simulink model "Model_Comparison_mks_landinglinear"  (R2022b)
settings: Solver=VariableStepAuto  StartTime=0.0  StopTime=4500  FixedStep=0.5  RelTol=1e-6
settings Model: Creator=Mitarbeiter  LastModifiedBy=Mitarbeiter

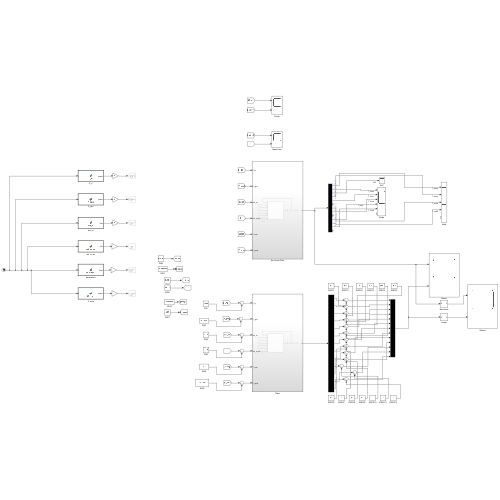
[thumbnail: Simulink's stored preview of the top-level diagram]
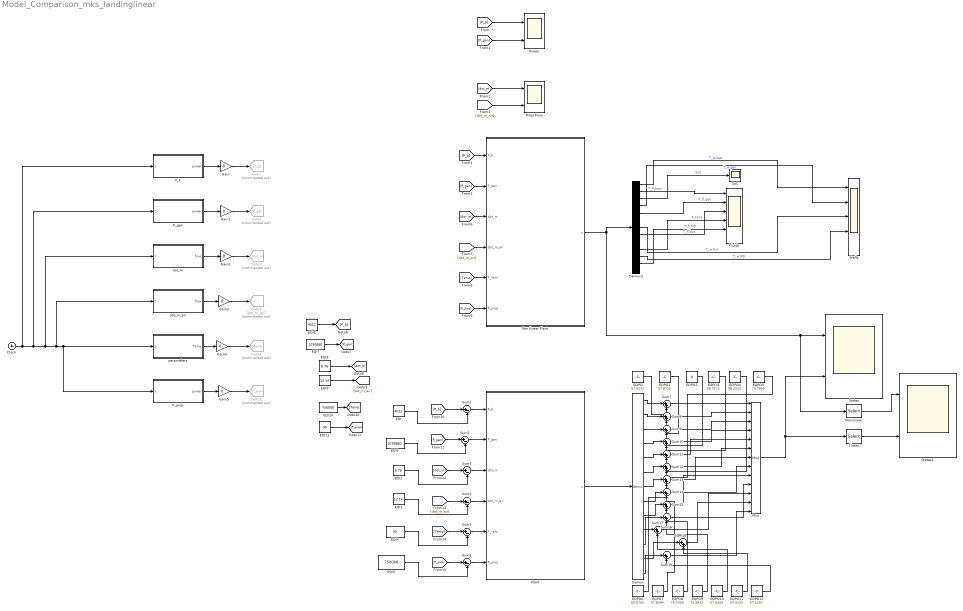
== system Model_Comparison_mks_landinglinear ==
  Clock : Clock
  Demux : Demux  Outputs=13
  Demux1 : Demux  Outputs=13
  EQI : Constant  Value=4012
  EQI1 : Constant  Value=1076880
  EQI10 : Constant  Value=750000
  EQI11 : Constant  Value=30
  EQI2 : Constant  Value=6.76
  EQI3 : Constant  Value=12.14
  EQI4 : Constant  Value=30
  EQI5 : Constant  Value=750000
  EQI6 : Constant  Value=4012
  EQI7 : Constant  Value=1076880
  EQI8 : Constant  Value=6.76
  EQI9 : Constant  Value=12.14
  EQPO : Constant  Value=57.9131
  EQPO1 : Constant  Value=57.8725
  EQPO10 : Constant  Value=57.8394
  EQPO11 : Constant  Value=57.3135
  EQPO12 : Constant  Value=57.1297
  EQPO2 : Constant  Value=0
  EQPO3 : Constant  Value=58.7172
  EQPO4 : Constant  Value=58.2512
  EQPO5 : Constant  Value=74.7995
  EQPO6 : Constant  Value=65.6701
  EQPO7 : Constant  Value=57.8394
  EQPO8 : Constant  Value=76.7055
  EQPO9 : Constant  Value=71.8433
  Fluids : Scope  NumInputPorts=6
  Gain{,1..5} (6 alike) : Gain  Gain=0
  Goto : Goto  Commented=on  GotoTag=P_b
  Goto1 : Goto  Commented=on  GotoTag=P_gen
  Goto2 : Goto  Commented=on  GotoTag=dot_m
  Goto3 : Goto  Commented=on  GotoTag=dot_m_air
  Goto4 : Goto  Commented=on  GotoTag=Temp
  Goto5 : Goto  Commented=on  GotoTag=P_prop
  Linear : Selector  InputPortWidth=13  IndexOptions=Index vector (dialog)  Indices=[1 2 3 4 5 6 7 8 9 10]  OutputSizes=1
  Mass Flow : Scope  NumInputPorts=2
  Mux : Mux  Inputs=13
  Non linear Plant : Subsystem
  Non-linear : Selector  InputPortWidth=13  IndexOptions=Index vector (dialog)  Indices=[1 2 3 4 5 6 7 8 9 10]  OutputSizes=1
  P_b : MATLAB Function  TreatAsAtomicUnit=on
  P_gen : MATLAB Function  TreatAsAtomicUnit=on
  P_prop : MATLAB Function  TreatAsAtomicUnit=on
  Plant : Subsystem
  Power : Scope  NumInputPorts=2
  SoC : Scope
  States : Scope  NumInputPorts=2
  States1 : Scope  NumInputPorts=2
  Sum{1..6} (6 alike) : Sum  Inputs=|+-
  Sum{7..19} (13 alike) : Sum  Inputs=|++
  Walls : Scope  NumInputPorts=5
  dot_m : MATLAB Function  TreatAsAtomicUnit=on
  dot_m_air : MATLAB Function  TreatAsAtomicUnit=on
  parameters : MATLAB Function  TreatAsAtomicUnit=on
  wires:
  Clock/1 -> P_b/1(t), P_gen/1(t), dot_m/1(t), dot_m_air/1(t), parameters/1(t), P_prop/1(t)
  Non linear Plant/1(x) -> Demux1/1, Non-linear/1, States/1
  Demux1/3 -> SoC/1  "SoC"
  Demux1/1 -> Walls/1  "T_w,batt"
  Demux1/2 -> Fluids/1  "T_fl,batt"
  Demux1/4 -> Walls/2  "T_w,gen"
  Demux1/5 -> Fluids/2  "T_fl,gen"
  Demux1/7 -> Walls/3  "T_w,bus"
  Demux1/8 -> Fluids/3  "T_fl,bus"
  Demux1/10 -> Fluids/4  "T_tank"
  Demux1/12 -> Fluids/5  "T_fl,MD"
  Demux1/11 -> Walls/4  "T_w,MD"
  dot_m/1(flow) -> Gain2/1
  P_gen/1(power) -> Gain1/1
  Plant/1(x) -> Demux/1
  Mux/1 -> States/2, Linear/1
  Non-linear/1 -> States1/1
  Linear/1 -> States1/2
  dot_m_air/1(flow) -> Gain3/1
  [P_b] -> Power/1
  [P_gen] -> Power/2
  [dot_m] -> Mass Flow/1
  [dot_m_air] -> Mass Flow/2
  P_b/1(power) -> Gain/1
  [P_b] -> Non linear Plant/1(P_b)
  [P_gen] -> Non linear Plant/2(P_gen)
  [dot_m] -> Non linear Plant/3(dot_m)
  [dot_m_air] -> Non linear Plant/4(dot_m_air)
  parameters/1(Temp) -> Gain4/1
  P_prop/1(power) -> Gain5/1
  [Temp] -> Non linear Plant/5(T_ram)
  [P_prop] -> Non linear Plant/6(P_prop)
  Sum2/1 -> Plant/1(P_b)
  [P_b] -> Sum2/1
  Sum1/1 -> Plant/2(P_gen)
  [dot_m] -> Sum3/1
  [P_gen] -> Sum1/1
  [dot_m_air] -> Sum4/1
  [Temp] -> Sum5/1
  [P_prop] -> Sum6/1
  Sum3/1 -> Plant/3(dot_m)
  Sum4/1 -> Plant/4(dot_m_air)
  Sum5/1 -> Plant/5(T_ram)
  Sum6/1 -> Plant/6(P_prop)
  EQI1/1 -> Sum1/2
  EQI/1 -> Sum2/2
  EQI2/1 -> Sum3/2
  EQI3/1 -> Sum4/2
  EQI4/1 -> Sum5/2
  EQI5/1 -> Sum6/2
  Demux/1 -> Sum7/1
  Demux/2 -> Sum8/1
  Demux/3 -> Sum9/1
  Demux/4 -> Sum10/1
  Demux/5 -> Sum11/1
  Demux/6 -> Sum12/1
  Demux/7 -> Sum13/1
  Demux/8 -> Sum14/1
  Demux/9 -> Sum15/1
  Demux/10 -> Sum16/1
  Demux/11 -> Sum17/1
  Demux/12 -> Sum18/1
  Demux/13 -> Sum19/1
  Sum7/1 -> Mux/1
  Sum8/1 -> Mux/2
  Sum9/1 -> Mux/3
  Sum10/1 -> Mux/4
  Sum11/1 -> Mux/5
  Sum12/1 -> Mux/6
  Sum13/1 -> Mux/7
  Sum14/1 -> Mux/8
  Sum15/1 -> Mux/9
  Sum16/1 -> Mux/10
  Sum17/1 -> Mux/11
  Sum18/1 -> Mux/12
  Sum19/1 -> Mux/13
  EQPO/1 -> Sum7/2
  EQPO1/1 -> Sum8/2
  EQPO2/1 -> Sum9/2
  EQPO3/1 -> Sum10/2
  EQPO4/1 -> Sum11/2
  EQPO5/1 -> Sum12/2
  EQPO6/1 -> Sum13/2
  EQPO7/1 -> Sum14/2
  EQPO8/1 -> Sum15/2
  EQPO9/1 -> Sum16/2
  EQPO10/1 -> Sum17/2
  EQPO11/1 -> Sum18/2
  EQPO12/1 -> Sum19/2
  Gain/1 -> Goto/1
  Gain1/1 -> Goto1/1
  Gain2/1 -> Goto2/1
  Gain3/1 -> Goto3/1
  Gain4/1 -> Goto4/1
  Gain5/1 -> Goto5/1
  EQI6/1 -> [P_b]
  EQI7/1 -> [P_gen]
  EQI8/1 -> [dot_m]
  EQI9/1 -> [dot_m_air]
  EQI10/1 -> [Temp]
  EQI11/1 -> [P_prop]

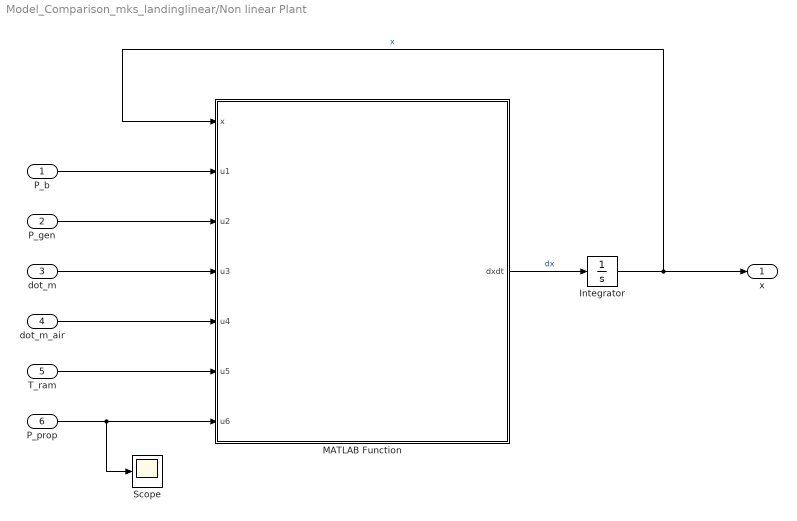
== system Model_Comparison_mks_landinglinear/Non linear Plant ==
  P_b : Inport
  P_gen : Inport  Port=2
  dot_m : Inport  Port=3
  dot_m_air : Inport  Port=4
  T_ram : Inport  Port=5
  P_prop : Inport  Port=6
  Integrator : Integrator  InitialCondition=[57.913; 57.872; 0; 58.717; 58.251; 74.799; 65.670; 57.839; 76.705; 71.843; 57.839; 57.313; 57.130]
  MATLAB Function : MATLAB Function  TreatAsAtomicUnit=on
  Scope : Scope
  x : Outport
  wires:
  MATLAB Function/1(dxdt) -> Integrator/1  "dx"
  Integrator/1 -> x/1, MATLAB Function/1(x)  "x"
  P_prop/1 -> Scope/1, MATLAB Function/7(u6)
  P_b/1 -> MATLAB Function/2(u1)
  P_gen/1 -> MATLAB Function/3(u2)
  dot_m/1 -> MATLAB Function/4(u3)
  dot_m_air/1 -> MATLAB Function/5(u4)
  T_ram/1 -> MATLAB Function/6(u5)

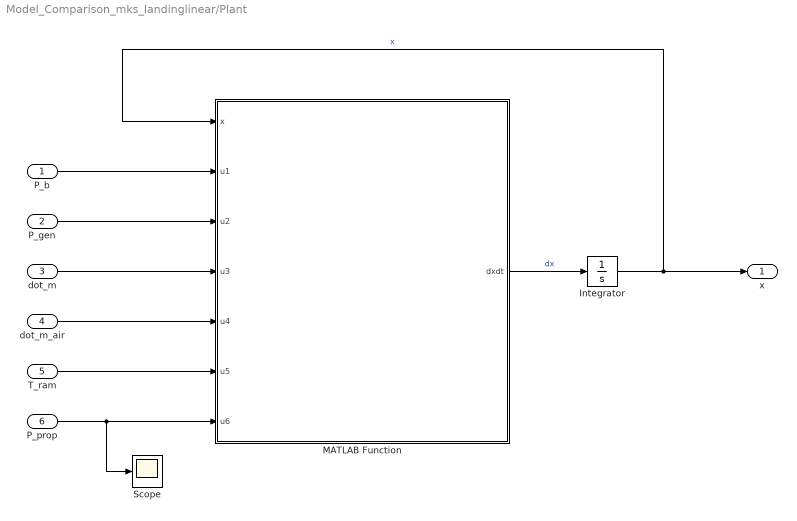
== system Model_Comparison_mks_landinglinear/Plant ==
  P_b : Inport
  P_gen : Inport  Port=2
  dot_m : Inport  Port=3
  dot_m_air : Inport  Port=4
  T_ram : Inport  Port=5
  P_prop : Inport  Port=6
  Integrator : Integrator  InitialCondition=[-27.9131; -27.8725; 0.9500; -28.7172; -28.2512; -44.7995; -35.6701; -27.8394; -46.7055; -41.8433; -27.8394; -27.3135; -27.1297];
  MATLAB Function : MATLAB Function  TreatAsAtomicUnit=on
  Scope : Scope
  x : Outport
  wires:
  MATLAB Function/1(dxdt) -> Integrator/1  "dx"
  Integrator/1 -> x/1, MATLAB Function/1(x)  "x"
  P_prop/1 -> Scope/1, MATLAB Function/7(u6)
  P_b/1 -> MATLAB Function/2(u1)
  P_gen/1 -> MATLAB Function/3(u2)
  dot_m/1 -> MATLAB Function/4(u3)
  dot_m_air/1 -> MATLAB Function/5(u4)
  T_ram/1 -> MATLAB Function/6(u5)

== matlab function Model_Comparison_mks_landinglinear/P_prop ==
  data: t input; power output
function power = P_prop(t)
    slope = 568.2;
    T_off = 60;
    cruise_t = 1380; % 23min
    landing_t = 3240; % 54min
    step = 1500e3;
    
    ramp1 = zeros(size(t));
    ramp1(t >= T_off) = -slope * (t(t >= T_off) - T_off);
    
    ramp2 = zeros(size(t));
    ramp2(t >= cruise_t) = slope * (t(t >= cruise_t) - cruise_t);
    
    ramp3 = zeros(size(t));
    ramp3(t >= landing_t) = -slope * (t(t >= landing_t) - landing_t);
    
    power = step + ramp1 + ramp2 + ramp3;
    power(power < 0) = 0;
   % power = 750000* ones(size(t));
end

== matlab function Model_Comparison_mks_landinglinear/Non linear Plant/MATLAB Function ==
  data: x input; dxdt output; u1 input; u2 input; u3 input; u4 input; u5 input; u6 input
function dxdt = fcn(x,u1,u2,u3,u4,u5,u6)

u = [u1;u2;u3;u4;u5;u6];

% Efficiencies
    d.e.eta_b = 0.9;
    d.e.eta_c = 0.93;
    d.e.eta_bus = 0.99;
    d.e.eta_m = 0.9;
    d.e.eta_i = 0.93;
    d.e.eta_g = 0.9;
    d.e.eta_r = 0.93;

    d.e.Batt_m = 833;   % Mass
    d.e.Batt_rho = 300; % Density

    cp_water = 4200;    % J/(kg.C) at 20C
    cp_fl = 2800;       % J/(kg.C) at 20C

    d.T.cp = 0.5 * cp_fl + 0.5 * cp_water; % Fluid specific heat capacity
    d.T.cp_air = 1006; % Air specific heat capacity

    d.HX.h_a = 10500;
    d.HX.h_b = 17500;
    d.HX.A_a = 60;
    d.HX.A_b = 103;

    d.CP.h = 8500;
    d.CP.A = 2.262;

    d.CP.A_MD = 3.534;
    masses = [70, 290, 630, 50, 210, 80, 330, 200, 90, 500, 130, 150, 70];

    C_batt = d.e.Batt_rho* masses(3)*3600; % kWs

    capacitance = d.T.cp * masses;
    
    capacitance(3) = C_batt;
    capacitance(13) = d.T.cp_air * masses(13);

    C = diag(capacitance);

    M = [1 -1 0 0 0 0 0 0 0 0 0 0 0 0 0;
         0 1 0 -1 0 1 0 0 0 0 0 0 0 0 0;
        -1 0 -1 0 0 0 0 0 0 0 0 0 0 0 0;
         0 0 0 0 -1 0 0 0 0 0 0 0 0 0 0;
         0 0 0 1 1 0 -1 0 0 0 0 0 0 0 0;
         0 0 0 0 0 0 0 -1 0 0 0 0 0 0 0;
         0 0 0 0 0 0 1 1 0 -1 0 0 0 0 0;
         0 0 0 0 0 -1 0 0 0 0 0 1 0 0 0;
         0 0 0 0 0 0 0 0 -1 0 0 0 0 0 0;
         0 0 0 0 0 0 0 0 1 1 -1 0 0 0 0;
         0 0 0 0 0 0 0 0 0 0 1 -1 -1 0 0;
         0 0 0 0 0 0 0 0 0 0 0 0 1 -1 0;
         0 0 0 0 0 0 0 0 0 0 0 0 0 1 -1;];

    D = [0 0 0 0;
         0 0 0 0;
         0 0 0 0;
         0 1 0 0;
         0 0 0 0;
         0 0 1 0;
         0 0 0 0;
         0 0 0 0;
         0 0 0 1;
         0 0 0 0;
         0 0 0 0;
         0 0 0 0;
         1 0 0 0;];

    P = [u(1)*(1-d.e.eta_b*d.e.eta_c)/(d.e.eta_b*d.e.eta_c);
         d.CP.h*d.CP.A*(x(1)-x(2));
         u(1);
         u(3)*d.T.cp*x(2);
         d.CP.h*d.CP.A*(x(4)-x(5));
         u(3)*d.T.cp*x(8);
         u(3)*d.T.cp*x(5);
         d.CP.h*d.CP.A*(x(6)-x(7));
         d.CP.h*d.CP.A_MD*(x(9)-x(10));
         u(3)*d.T.cp*x(7);
         u(3)*d.T.cp*x(10);
         u(3)*d.T.cp*x(11);
         d.HX.h_a*d.HX.A_a*(x(11)-x(12));
         d.HX.h_b*d.HX.A_b*(x(12)-x(13));
         u(4)*d.T.cp_air*x(13)];

    P_in = [u(4)*d.T.cp_air*u(5);
            u(6)*(1-d.e.eta_bus)/(d.e.eta_m*d.e.eta_i);
            (1-d.e.eta_g*d.e.eta_r)*u(2);
            u(6)*(1-d.e.eta_m*d.e.eta_i)/(d.e.eta_m*d.e.eta_i);];

    x_dot_n = C \ (M * P + D * P_in);

dxdt = x_dot_n;

== matlab function Model_Comparison_mks_landinglinear/P_b ==
  data: t input; power output
function power = P_b(t)
    % Define the power values vector
    power_values = [541728.972461324, 525434.547259656, 484698.484257782, ...
                    443962.421182278, 403226.358083855, 362490.295190934, ...
                    321754.232292711, 281018.169380235, 240282.106417171, ...
                    199546.043463649, 158809.980492022, 118073.917524794, ...
                    77337.8545513178, 36601.7915815174, 4012.94120061964, ...
                    4012.94120060897, 4012.94120058611, 4012.94120055903, ...
                    4012.94120053569, 4012.94120052215, 4012.94120051169, ...
                    4012.94120050506, 4012.94120050103, 4012.94120049878, ...
                    4012.94120049977, 4012.94120050145, 4012.94120050538, ...
                    4012.94120051198, 4012.94120052045, 4012.94120053546, ...
                    4012.94120055757, 4012.94120058035, 4012.94120057094, ...
                    9.73312208790910e-10, -3.25790856001986e-10, ...
                    -7.33764827360896e-10, -3.22870604452897e-11, ...
                    -2.89901400312855e-11, -6.19593223381754e-11, ...
                    -4.77143652162351e-10, 3.07295526727322e-10, ...
                    -5.97594860992170e-10, 7.70455739254353e-10, ...
                    -4.62243586863996e-11, 65143.2880368747];

    % Define the corresponding time vector (every 10 seconds from 0 to 4500)
    time_vector = 1:100:4500;

    % Check if input t is within the range of 0 to 4500
    if t < 0 || t > 4500
        error('Input time t must be within the range 0 to 4500 seconds.');
    end

    % Create the spline interpolation function
    spline_fit = spline(time_vector, power_values);

    % Evaluate the spline at the desired continuous time t
    power = ppval(spline_fit, t);

%     power = 4012* ones(size(t));
end

== matlab function Model_Comparison_mks_landinglinear/P_gen ==
  data: t input; power output
function power = P_gen(t)
  
    power_values = [1560823.08194895	1546158.09929008	1509495.64264034	1472833.18607241	1436170.72952995	1399508.27275915	1362845.81599425	1326183.35924518	1289520.90255232	1252858.44584885	1216195.98916551	1179533.53247727	1142871.07579598	1106208.61911061	1076878.65376792	1076878.65376794	1076878.65376796	1076878.65376799	1076878.65376802	1076878.65376803	1076878.65376804	1076878.65376805	1076878.65376806	1076878.65376806	1076878.65376806	1076878.65376806	1076878.65376805	1076878.65376804	1076878.65376803	1076878.65376802	1076878.65376799	1076878.65376797	1076878.65376798	1032182.62799974	950257.879125699	868333.130251657	786408.381377613	704483.632503570	622558.883629528	540634.134755485	458709.385881442	376784.637007400	294859.888133355	212935.139259313	58628.9592331873];
 % Define the corresponding time vector (every 10 seconds from 0 to 4500)
    time_vector = 1:100:4500;

    % Check if input t is within the range of 0 to 4500
    if t < 0 || t > 4500
        error('Input time t must be within the range 0 to 4500 seconds.');
    end

    % Create the spline interpolation function
    spline_fit = spline(time_vector, power_values);

    % Evaluate the spline at the desired continuous time t
    power = ppval(spline_fit, t);

% power = 1076880* ones(size(t));
end

== matlab function Model_Comparison_mks_landinglinear/dot_m_air ==
  data: t input; flow output
function flow = dot_m_air(t)
    % Define the power values vector
    power_values = [0.370775472872228	4.14655917085228	10.2236066715828	15.9335661862365	19.0351731908349	16.9149763039733	13.1623042033400	10.7569435504486	8.94905877526484	7.51589529502896	6.36393337822089	5.39660249912924	4.60743235399543	4.39417963045294	4.45647923355531	4.36949731785185	4.31573725145724	4.26746478317914	4.22732179826729	4.19595415374334	4.17143491891122	4.15169555274063	4.13523300363972	4.12099504031059	4.10816091872904	4.09600581489035	4.08381103149970	4.07079463660703	4.05616667450225	4.03954164705557	4.02160559806096	4.00355147248531	3.98237533346872	3.81444977989844	3.58043631849297	3.43750882096772	3.44017594340288	3.48343898919501	3.38952732636595	3.08055145207970	2.48510068273254	1.52973911636135	0.577892294612315	0.0671525631123886	1.01083847375133e-34];

    % Define the corresponding time vector (every 10 seconds from 0 to 4500)
    time_vector = 1:100:4500;

    % Check if input t is within the range of 0 to 4500
    if t < 0 || t > 4500
        error('Input time t must be within the range 0 to 4500 seconds.');
    end

    % Create the spline interpolation function
    spline_fit = spline(time_vector, power_values);

    % Evaluate the spline at the desired continuous time t
    flow = ppval(spline_fit, t);
%     flow = 12.14* ones(size(t));
end

== matlab function Model_Comparison_mks_landinglinear/dot_m ==
  data: t input; flow output
function flow = dot_m(t)
    % Define the power values vector
    power_values = [0.904165131160427	1.62335959482857	1.97415345554372	2.87737856692485	3.93386755649844	4.17049006426838	3.96224826445125	3.84633136696794	3.73843209854831	3.62816620139765	3.51470105395037	3.39795514134232	3.27785630468602	3.15345777233773	3.04616198439548	3.03635175832522	2.98312074354866	2.91947217209040	2.86878591164222	2.83212849923799	2.80518126603719	2.78469068203536	2.76888505493890	2.75675815114367	2.74763217287481	2.74096591488524	2.73636304275517	2.73354386559958	2.73235420493226	2.73274273164412	2.73475441155951	2.73847704472223	2.74398498698495	2.64313697414983	2.45549965647436	2.26040185709996	2.23930438794837	1.99924539905101	1.61176185199414	1.31895743051123	1.30916014023536	1.07782805041202	0.848496416787671	0.620762639063214	-5.77778983316171e-34];

    % Define the corresponding time vector (every 10 seconds from 0 to 4500)
    time_vector = 1:100:4500;

    % Check if input t is within the range of 0 to 4500
    if t < 0 || t > 4500
        error('Input time t must be within the range 0 to 4500 seconds.');
    end

    % Create the spline interpolation function
    spline_fit = spline(time_vector, power_values);

    % Evaluate the spline at the desired continuous time t
    flow = ppval(spline_fit, t);

%     flow = 6.76* ones(size(t));
end

== matlab function Model_Comparison_mks_landinglinear/Plant/MATLAB Function ==
  data: x input; dxdt output; u1 input; u2 input; u3 input; u4 input; u5 input; u6 input
function dxdt = fcn(x,u1,u2,u3,u4,u5,u6)

u = [u1;u2;u3;u4;u5;u6];

 % Extract control inputs and disturbances from u
    u1 = u(1);  % Control input 1
    u2 = u(2);  % Control input 2
    u3 = u(3);  % Control input 3
    u4 = u(4);  % Control input 4
    xs = u(5);  % Disturbance related to xs
    xt = u(6);  % Disturbance related to xt

x = [x(1:2); x(4:end)];
%% A Matrix 
 
A = [-19227/245000, 19227/245000, 0, 0, 0, 0, 0, 0, 0, 0, 0, 0; 663/35000, -67399/2030000, 0, 0, 0, 0, 827/58000, 0, 0, 0, 0, 0; 0, 0, -19227/175000, 19227/175000, 0, 0, 0, 0, 0, 0, 0, 0; 0, 827/42000, 6409/245000, -67399/1470000, 0, 0, 0, 0, 0, 0, 0, 0; 0, 0, 0, 0, -19227/280000, 19227/280000, 0, 0, 0, 0, 0, 0; 0, 0, 0, 827/66000, 6409/385000, -67399/2310000, 0, 0, 0, 0, 0, 0; 0, 0, 0, 0, 0, 0, -827/40000, 0, 0, 827/40000, 0, 0; 0, 0, 0, 0, 0, 0, 0, -10013/105000, 10013/105000, 0, 0, 0; 0, 0, 0, 0, 0, 827/100000, 0, 30039/1750000, -89023/3500000, 0, 0, 0; 0, 0, 0, 0, 0, 0, 0, 0, 827/26000, -36827/26000, 18/13, 0; 0, 0, 0, 0, 0, 0, 0, 0, 0, 6/5, -139/30, 103/30; 0, 0, 0, 0, 0, 0, 0, 0, 0, 0, 12875/503, -113193957/4401250];

B = [163/205065000, 0, 0, 0; 0, 0, -2281348/702581985, 0; 0, 0, 0, 0; 0, 0, -6274/11305917, 0; 0, 163/280000000, 0, 0; 0, 0, -5830021/955185000, 0; 0, 0, 0, 0; 0, 0, 0, 0; 0, 0, -511331/134594250, 0; 0, 0, 12045384577/314950545000, 0; 0, 0, 0, 0; 0, 0, 0, -8752431102689/31504253130000];

P0 = [0; 570337/42477750; 0; 3137/1367100; 0; 5830021/231000000; 0; 0; 511331/32550000; -12045384577/76167000000; 0; 8752431102689/3683846250000];

E = [0, 0; 0, 0; 1/14647500, 0; 0, 0; 0, 0; 0, 0; 0, 0; 163/263655000, 0; 0, 0; 0, 0; 0, 0; 0, 1/70420];

    u = [u1; u2; u3; u4];
    P_s = u4*1006*xs;
x_dot = A * x + B * u + E * [xt;P_s] + P0;

% B_cap is in Wh; to convert it into Ws its multiplied by 3600
% B_cap is actually battery density in Wh/kg (here 300) multiplied ...
% by mass of battery (here 630 kg)
% 1000/837 comes after inputting values for eta_b, eta_c in the equation!

SoC_equation = -1000/(837*300*630*3600)*u1; 

    dxdt = [x_dot(1:2); SoC_equation; x_dot(3:end)];

== matlab function Model_Comparison_mks_landinglinear/parameters ==
  data: t input; Temp output
function Temp  = parameters(t)
    %% Calculates aircraft altitude in ft and m

    T_off = 60;
    cruise_t = 1380;
    landing_t = 3240;
    final_t = 4500;

    slope1 = 0.25/T_off; % 0.25 / 1
    slope2 = (0.4 - 0.25) / (cruise_t - T_off);
    slope3 = (0.25 - 0.4) / (final_t - landing_t);

    ramp = zeros(size(t));
    ramp(t <= T_off) = slope1 * t(t <= T_off);
    
    ramp1 = zeros(size(t));
    ramp1(t > T_off & t < cruise_t) = slope2 * (t(t > T_off & t < cruise_t) - T_off) + 0.25;
    
    ramp2 = zeros(size(t));
    ramp2(t >= cruise_t & t <= landing_t) = 0.4;
    
    ramp3 = zeros(size(t));
    ramp3(t > landing_t & t <= 4500) = slope3 * (t(t > landing_t & t <= 4500) - landing_t) + 0.4;
    
    ramp4 = zeros(size(t));
    ramp4(t > 4500) = slope3 * (t(t > 4500) - 4500) + 0.25;
    
    Speed = ramp + ramp1 + ramp2 + ramp3 + ramp4;

    %% T_ram calculations
    r_slope1 = 0;
    r_slope2 = (-35 - 30) / (1380 - 60);
    r_slope3 = 0;
    
    r_slope5 = (30 - (-35)) / (4500 - 3240);
    
    Gamma = 1.4;
    
    ramp = zeros(size(t));
    ramp(t <= T_off) = r_slope1 * t(t <= T_off) + 30;
    
    ramp1 = zeros(size(t));
    ramp1(t > T_off & t < cruise_t) = r_slope2 * (t(t > T_off & t < cruise_t) - T_off) + 30;
    
    ramp2 = zeros(size(t));
    ramp2(t >= cruise_t & t <= landing_t) = -35;
    
    ramp3 = zeros(size(t));
    ramp3(t > landing_t & t <= 4500) = r_slope5 * (t(t > landing_t & t <= 4500) - landing_t) - 35;
    
    ramp4 = zeros(size(t));
    ramp4(t > 4500) = r_slope3 * (t(t > 4500) - 4500) + 30;
    
    T_amp = ramp + ramp1 + ramp2 + ramp3 + ramp4;

     Temp = T_amp.*(1+Speed.^2 * ((Gamma-1)/2));
%     Temp = 30 * ones(size(t));

end
